simulink model "QuadRotor_PID_Simulink3d"  (R2014a)
settings: Solver=ode45  StartTime=0.0  StopTime=inf
PreLoadFcn:
  | load CommandsBus
model workspace (MAT data in the model file):
  thrustConstant = Simulink.Parameter
  thrustConstant.Value = -0.001
  thrustConstant.Description = '-0.004'
  thrustConstant.DataType = 'double'
  torqueConstant = Simulink.Parameter
  torqueConstant.Value = -4e-05
  torqueConstant.DataType = 'auto'
undefined symbols (not defined in the file or in its folder): X, Y, Z
libraries: sm_lib x829, nesl_utility x156, simulink x12, fl_lib x4, vrlib x4, aerolibtransform2 x1
(part 1 of 18)
settings Model: Creator=Leonardo  LastModifiedBy=jsustare
settings DataIOCC: OutputTimes=(1:900)*1/30
settings OptimizationCC: BlockReduction=off
settings DebuggingCC: UnderspecifiedInitializationDetection=Classic
settings ExplorerConfigSet: InternalSimMechanicsExplorerSettings="<ExplorerConfiguration><canonicalview>default</canonicalview><TilePanel><TileInfo><Tiles Columns=\"1\" Count=\"1\" Rows=\"1\"><Column Left=\"2\" Weight=\"1\"/><Column Left=\"1104\"/><Row Top=\"2\" Weight=\"1\"/><Row Top=\"593\"/><Tile Height=\"1\" Width=\"1\" X=\"0\" Y=\"0\"/></Tiles></TileInfo><SceneInfo><SceneViewer><BGColor><R>0.60000002384185791</R><G>0.60000002384185791</G><B>0.60000002384185791</B></BGColor><Camera><Position><X>6.7360474591593813e-05</X><Y>0.35928378687683804</Y><Z>0.81921140974164575</Z></Position><Center><X>6.7360474591593813e-05</X><Y>0.35928378687683804</Y><Z>0</Z></Center><Up><X>0</X><Y>1</Y><Z>-0</Z></Up><Left>-0.51821660457900831</Left><Right>0.51821660457900831</Right><Bottom>-0.41561021241290713</Bottom><Top>0.41561021241290713</Top></Camera></SceneViewer></SceneInfo></TilePanel></ExplorerConfiguration>"

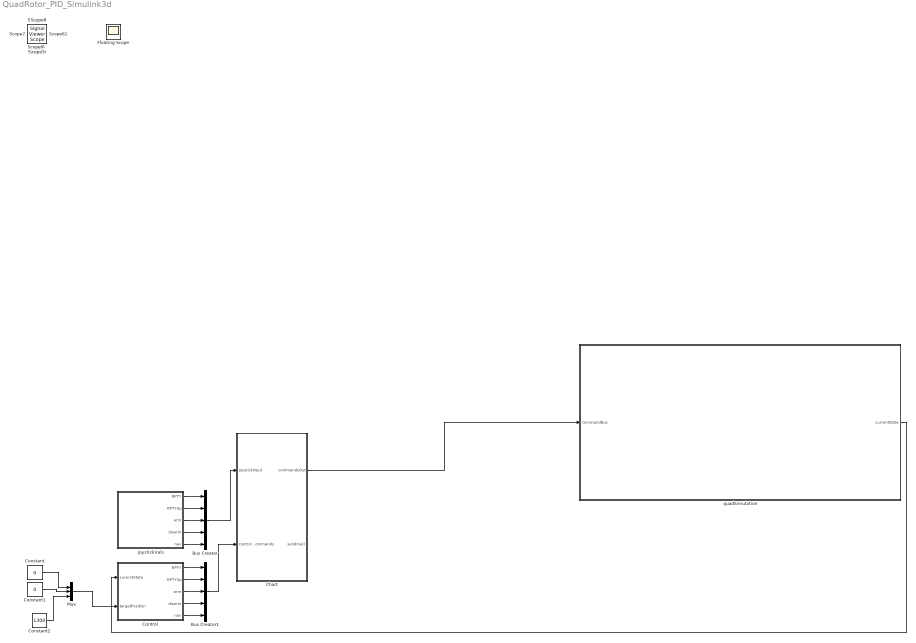
== system QuadRotor_PID_Simulink3d ==
  Bus Creator : BusCreator  Inputs=5
  Bus Creator1 : BusCreator  Inputs=5  OutDataTypeStr=Bus: CommandsBus
  Chart : Stateflow chart  TreatAsAtomicUnit=on
  Constant : Constant  Value=0
  Constant1 : Constant  Value=0
  Constant2 : Constant  Value=1300
  Control : Subsystem
  Mux : Mux  Inputs=3
  joystickVals : Subsystem
  quadSimulation : Subsystem
  Floating Scope : Scope
      settings: Floating=on  YMin=-0.125  YMax=0.15  SaveName=ScopeData8
  Scope{,1..4} (5 alike) : SignalViewerScope  IOType=viewer  RefreshTime=0.035000
      Scope settings: YMin=-0.7  YMax=0.1  SaveName=ScopeData4
      Scope1 settings: YMin=5.81481  YMax=6.42689
      Scope3 settings: YMin=-2.5  YMax=20  SaveName=ScopeData2
      Scope4 settings: YMin=0.0225  YMax=0.05  SaveName=ScopeData3
  Scope10 : SignalViewerScope  IOType=viewer  NumInputPorts=3  LegendLocations=|  RefreshTime=0.035000
      | 0.58116     0.90774     0.17375    0.026284
      | 0.69749     0.61398     0.23192    0.026284
      | 0.67959         0.3     0.24981    0.026284
      settings: ShowLegends=on  YMin=-0.09~-400~-1  YMax=0.1~450~1  SaveName=ScopeData10
  Scope11 : SignalViewerScope  IOType=viewer  NumInputPorts=3  RefreshTime=0.035000
      settings: YMin=-0.5~-750~-1  YMax=9.5~750~1  SaveName=ScopeData11
  Scope5 : SignalViewerScope  IOType=viewer  NumInputPorts=2  RefreshTime=0.035000
      settings: YMin=-55~-5  YMax=5~5  SaveName=ScopeData5
  Scope6 : SignalViewerScope  IOType=viewer  NumInputPorts=4  RefreshTime=0.035000
      settings: YMin=-35~-35~-550~-4  YMax=10~10~50~2  SaveName=ScopeData9
  Scope7 : SignalViewerScope  IOType=viewer  NumInputPorts=3  RefreshTime=0.035000
      settings: YMin=-0.1~-10~0  YMax=1.1~10~1  SaveName=ScopeData6
  Scope8 : SignalViewerScope  IOType=viewer  NumInputPorts=2  RefreshTime=0.035000
      settings: YMin=-125~-10  YMax=150~12.5  SaveName=ScopeData7
  Scope9 : SignalViewerScope  IOType=viewer  NumInputPorts=3  RefreshTime=0.035000
      settings: YMin=-0.1~-10~0  YMax=1.1~10~1  SaveName=ScopeData8
  wires:
  joystickVals/4(disarm) -> Bus Creator/4
  joystickVals/3(arm) -> Bus Creator/3
  joystickVals/5(nav) -> Bus Creator/5
  Bus Creator/1 -> Chart/1(joystickInput)
  Control/5(nav) -> Bus Creator1/5
  Control/4(disarm) -> Bus Creator1/4
  Control/3(arm) -> Bus Creator1/3
  Control/2(RPTYUp) -> Bus Creator1/2
  Control/1(RPTY) -> Bus Creator1/1
  Bus Creator1/1 -> Chart/2(controlCommands)
  joystickVals/1(RPTY) -> Bus Creator/1
  joystickVals/2(RPTYUp) -> Bus Creator/2
  Chart/1(commandsOut) -> quadSimulation/1(commandBus)
  quadSimulation/1(currentState) -> Control/1(curerntState)
  Constant/1 -> Mux/1
  Constant1/1 -> Mux/2
  Constant2/1 -> Mux/3
  Mux/1 -> Control/2(targetPosition)

== system QuadRotor_PID_Simulink3d/Control ==
  curerntState : Inport
  targetPosition : Inport  Port=2
  Band-Limited White Noise : simulink/Sources/Band-Limited White Noise  Cov=0.00005  Ts=0.1  seed=[23341]
  Band-Limited White Noise1 : simulink/Sources/Band-Limited White Noise  Cov=0.00005  Ts=0.1  seed=[23341]
  Band-Limited White Noise2 : simulink/Sources/Band-Limited White Noise  Cov=0.00005  Ts=0.1  seed=[23341]
  Constant : Constant  OutDataTypeStr=boolean
  Demux : Demux  Outputs=6
  Detect Change : simulink/Logic and Bit Operations/Detect Change  vinit=0  InputProcessing=Inherited  OutDataTypeStr=boolean
  Logical Operator : Logic  Operator=OR  Inputs=1  AllPortsSameDT=off  OutDataTypeStr=boolean
  Mux : Mux
  Sum : Sum  Inputs=|++
  Sum1 : Sum  Inputs=|++
  Sum2 : Sum  Inputs=|++
  failsafes : Subsystem
  positionControl : Subsystem
  RPTY : Outport
  RPTYUp : Outport  Port=2
  arm : Outport  Port=3
  disarm : Outport  Port=4
  nav : Outport  Port=5
  wires:
  Demux/5 -> Sum/2
  Demux/6 -> Sum1/2
  Demux/3 -> Sum2/2
  positionControl/1(R) -> Mux/1
  positionControl/2(P) -> Mux/2
  positionControl/4(Thrust) -> Mux/3
  positionControl/3(targetYaw) -> Mux/4
  Mux/1 -> Detect Change/1, RPTY/1
  Detect Change/1 -> Logical Operator/1
  Logical Operator/1 -> RPTYUp/1
  Constant/1 -> nav/1
  targetPosition/1 -> positionControl/4(targetPos)
  failsafes/1(arm) -> arm/1
  failsafes/2(disarm) -> disarm/1
  curerntState/1 -> Demux/1
  Band-Limited White Noise/1 -> Sum/1
  Sum/1 -> positionControl/1(X)
  Band-Limited White Noise1/1 -> Sum1/1
  Sum1/1 -> positionControl/2(Y)
  Band-Limited White Noise2/1 -> Sum2/1
  Sum2/1 -> positionControl/3(Heading)

== system QuadRotor_PID_Simulink3d/joystickVals ==
  Constant1 : Constant  Value=0  OutDataTypeStr=boolean
  Constant2 : Constant  Value=0  OutDataTypeStr=boolean
  Constant3 : Constant  Value=1500
  Constant4 : Constant  Value=1500
  Constant5 : Constant  Value=1059
  Constant6 : Constant  Value=1500
  Constant7 : Constant  OutDataTypeStr=boolean
  Detect Change : simulink/Logic and Bit Operations/Detect Change  vinit=0  InputProcessing=Inherited  OutDataTypeStr=boolean
  Logical Operator : Logic  Operator=OR  Inputs=1  AllPortsSameDT=off  OutDataTypeStr=boolean
  Mux : Mux
  RPTY : Outport
  RPTYUp : Outport  Port=2
  arm : Outport  Port=3
  disarm : Outport  Port=4
  nav : Outport  Port=5
  wires:
  Constant3/1 -> Mux/2
  Constant4/1 -> Mux/1
  Constant5/1 -> Mux/3
  Constant6/1 -> Mux/4
  Mux/1 -> RPTY/1, Detect Change/1  "RPTY"
  Detect Change/1 -> Logical Operator/1
  Logical Operator/1 -> RPTYUp/1  "RPTYUp"
  Constant1/1 -> arm/1  "arm"
  Constant2/1 -> disarm/1  "disarm"
  Constant7/1 -> nav/1  "nav"

== system QuadRotor_PID_Simulink3d/quadSimulation ==
  note: Pitch (Motor A,C)
      | Roll (Motor B,D)
      | Altitude(A,B,C,D)
      | Yaw (Unbalance A/C B/D)
  commandBus : Inport
  Controller : Subsystem
  Demux : Demux
  GetErrors : Subsystem
  Mux : Mux  Inputs=6
  Mux2 : Mux
  Plant_Quad_Base : Subsystem  Variant=on  OverrideUsingVariant=Quad_6DOF
  Rate Transition : RateTransition
  Scope6 : Scope  NumInputPorts=4
      settings: YMin=-5~-5~-5~-5  YMax=5~5~5~5  SaveName=ScopeData6
  SpdMin2Rotors : Constant  Value=0.058
  Vizualize Signals : Subsystem
  Vizualize Simulink 3d : Subsystem
  converting : Subsystem
  currentState : Outport
  wires:
  Plant_Quad_Base/1(Roll) -> Mux/1  "Roll"
  Plant_Quad_Base/2(Pitch) -> Mux/2  "Pitch"
  Plant_Quad_Base/3(Yaw) -> Mux/3  "Yaw"
  Plant_Quad_Base/4(Altitude) -> Mux/4  "Altitude"
  Controller/2(Act_B) -> Plant_Quad_Base/2(spdMotorB)
  Controller/3(Act_C) -> Plant_Quad_Base/3(spdMotorC)
  Controller/1(Act_A) -> Plant_Quad_Base/1(spdMotorA)
  Controller/4(Act_D) -> Plant_Quad_Base/4(spdMotorD)
  SpdMin2Rotors/1 -> Controller/1(Ref_Spd_Min)
  Demux/1 -> Scope6/1, Controller/2(Err_Roll)  "Err_Roll"
  Demux/2 -> Scope6/2, Controller/3(Err_Pitch)  "Err_Pitch"
  Demux/3 -> Scope6/3, Controller/4(Err_Yaw)  "Err_Yaw"
  Demux/4 -> Scope6/4, Controller/5(Err_Alt)  "Err_Alt"
  Plant_Quad_Base/5(X) -> Mux/5  "X"
  Plant_Quad_Base/6(Y) -> Mux/6  "Y"
  Rate Transition/1 -> GetErrors/1(References)
  GetErrors/1(Errors) -> Demux/1
  Mux2/1 -> Rate Transition/1
  Mux/1 -> GetErrors/2(Outputs), currentState/1
  commandBus/1 -> converting/1(In1)
  converting/1(Out1) -> Mux2/1
  converting/2(Out2) -> Mux2/2
  converting/3(Out3) -> Mux2/3
  converting/4(Out4) -> Mux2/4

== system QuadRotor_PID_Simulink3d/Control/failsafes ==
  Constant1 : Constant  Value=0  OutDataTypeStr=boolean
  arm : Outport
  disarm : Outport  Port=2
  wires:
  Constant1/1 -> disarm/1, arm/1

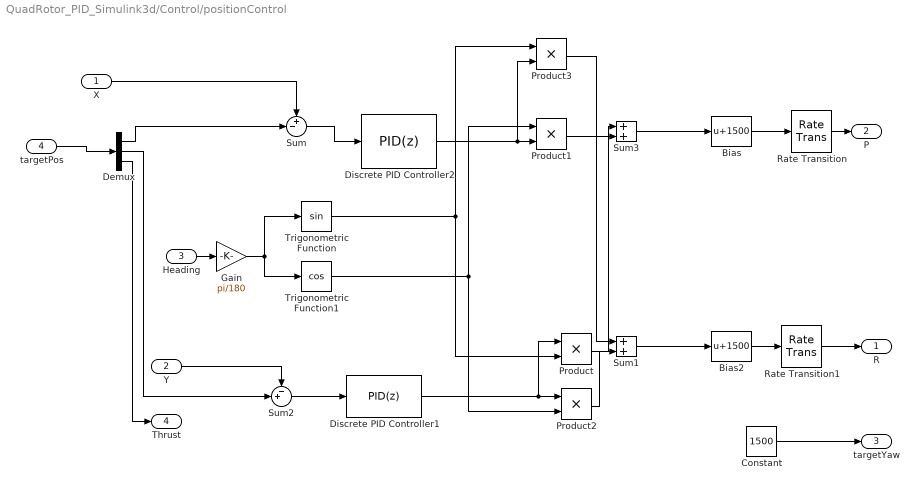
== system QuadRotor_PID_Simulink3d/Control/positionControl ==
  X : Inport
  Y : Inport  Port=2
  Heading : Inport  Port=3
  targetPos : Inport  Port=4
  Bias : Bias  Bias=1500
  Bias2 : Bias  Bias=1500
  Constant : Constant  Value=1500
  Demux : Demux  Outputs=3
  Discrete PID Controller1 : simulink/Continuous/PID Controller  Controller=PID  TimeDomain=Discrete-time  SampleTime=0.1  IntegratorMethod=Trapezoidal  FilterMethod=Trapezoidal  Form=Parallel  P=300  I=0  D=250  N=100  InitialConditionSource=internal  InitialConditionForIntegrator=0  InitialConditionForFilter=0  ExternalReset=none  ZeroCross=off  LimitOutput=on  UpperSaturationLimit=500  LowerSaturationLimit=-500  LinearizeAsGain=off  AntiWindupMode=clamping  Kb=1  TrackingMode=off  Kt=1  PParamMin=[]  PParamMax=[]  IParamMin=[]  IParamMax=[]  DParamMin=[]  DParamMax=[]  NParamMin=[]  NParamMax=[]  KbParamMin=[]  KbParamMax=[]  KtParamMin=[]  KtParamMax=[]  POutMin=[]  POutMax=[]  IOutMin=[]  IOutMax=[]  DOutMin=[]  DOutMax=[]  NOutMin=[]  NOutMax=[]  KbOutMin=[]  KbOutMax=[]  KtOutMin=[]  KtOutMax=[]  IntegratorOutMin=[]  IntegratorOutMax=[]  FilterOutMin=[]  FilterOutMax=[]  SumOutMin=[]  SumOutMax=[]  SumI1OutMin=[]  SumI1OutMax=[]  SumI2OutMin=[]  SumI2OutMax=[]  SumI3OutMin=[]  SumI3OutMax=[]  SumDOutMin=[]  SumDOutMax=[]  SaturationOutMin=[]  SaturationOutMax=[]  IntegratorContinuousStateAttributes=''  IntegratorStateMustResolveToSignalObject=off  IntegratorRTWStateStorageClass=Auto  FilterContinuousStateAttributes=''  FilterStateMustResolveToSignalObject=off  FilterRTWStateStorageClass=Auto
  Discrete PID Controller2 : simulink/Continuous/PID Controller  Controller=PID  TimeDomain=Discrete-time  SampleTime=0.1  IntegratorMethod=Trapezoidal  FilterMethod=Trapezoidal  Form=Parallel  P=300  I=0  D=250  N=100  InitialConditionSource=internal  InitialConditionForIntegrator=0  InitialConditionForFilter=0  ExternalReset=none  ZeroCross=off  LimitOutput=on  UpperSaturationLimit=500  LowerSaturationLimit=-500  LinearizeAsGain=off  AntiWindupMode=clamping  Kb=1  TrackingMode=off  Kt=1  PParamMin=[]  PParamMax=[]  IParamMin=[]  IParamMax=[]  DParamMin=[]  DParamMax=[]  NParamMin=[]  NParamMax=[]  KbParamMin=[]  KbParamMax=[]  KtParamMin=[]  KtParamMax=[]  POutMin=[]  POutMax=[]  IOutMin=[]  IOutMax=[]  DOutMin=[]  DOutMax=[]  NOutMin=[]  NOutMax=[]  KbOutMin=[]  KbOutMax=[]  KtOutMin=[]  KtOutMax=[]  IntegratorOutMin=[]  IntegratorOutMax=[]  FilterOutMin=[]  FilterOutMax=[]  SumOutMin=[]  SumOutMax=[]  SumI1OutMin=[]  SumI1OutMax=[]  SumI2OutMin=[]  SumI2OutMax=[]  SumI3OutMin=[]  SumI3OutMax=[]  SumDOutMin=[]  SumDOutMax=[]  SaturationOutMin=[]  SaturationOutMax=[]  IntegratorContinuousStateAttributes=''  IntegratorStateMustResolveToSignalObject=off  IntegratorRTWStateStorageClass=Auto  FilterContinuousStateAttributes=''  FilterStateMustResolveToSignalObject=off  FilterRTWStateStorageClass=Auto
  Gain : Gain  Gain=pi/180
  Product{,1..3} (4 alike) : Product
  Rate Transition : RateTransition
  Rate Transition1 : RateTransition
  Sum : Sum  Inputs=+-|
  Sum1 : Sum
  Sum2 : Sum  Inputs=-+|
  Sum3 : Sum
  Trigonometric Function : Trigonometry
  Trigonometric Function1 : Trigonometry  Operator=cos
  R : Outport
  P : Outport  Port=2
  targetYaw : Outport  Port=3
  Thrust : Outport  Port=4
  wires:
  Sum/1 -> Discrete PID Controller2/1
  Heading/1 -> Gain/1
  Gain/1 -> Trigonometric Function/1, Trigonometric Function1/1
  Discrete PID Controller1/1 -> Product/1, Product2/1
  Trigonometric Function/1 -> Product/2, Product3/1
  Discrete PID Controller2/1 -> Product3/2, Product1/2
  Trigonometric Function1/1 -> Product2/2, Product1/1
  Product1/1 -> Sum3/2
  Product2/1 -> Sum1/2
  Sum3/1 -> Bias/1
  Product3/1 -> Sum1/1
  targetPos/1 -> Demux/1
  Demux/1 -> Sum/2
  Constant/1 -> targetYaw/1
  Rate Transition/1 -> P/1
  Rate Transition1/1 -> R/1
  Bias/1 -> Rate Transition/1
  Demux/3 -> Thrust/1
  Product/1 -> Sum3/1
  Sum1/1 -> Bias2/1
  Bias2/1 -> Rate Transition1/1
  Sum2/1 -> Discrete PID Controller1/1
  Demux/2 -> Sum2/2
  Y/1 -> Sum2/1
  X/1 -> Sum/1

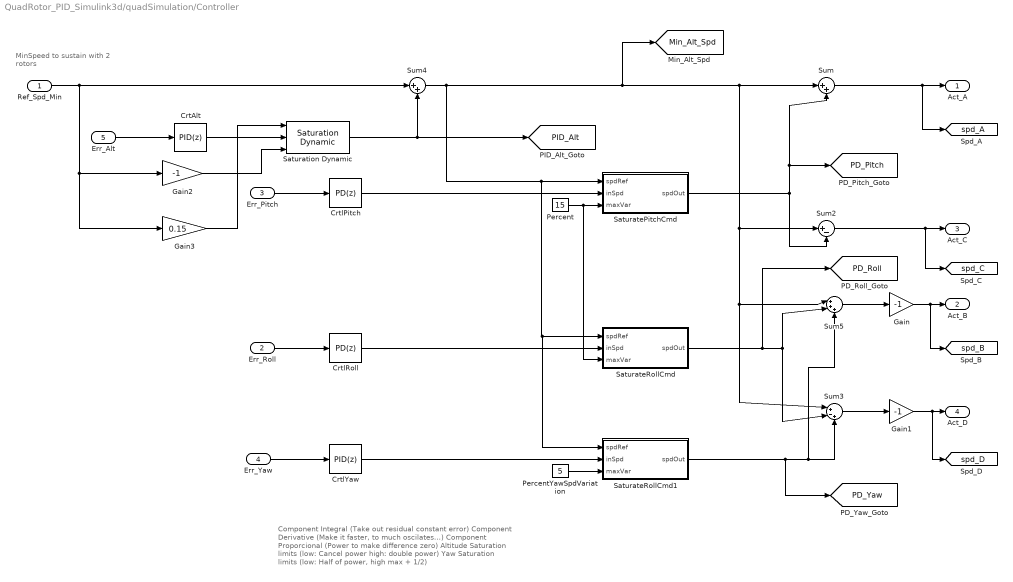
== system QuadRotor_PID_Simulink3d/quadSimulation/Controller ==
  note: MinSpeed to sustain with 2
      | rotors
  note: Component Integral (Take out residual constant error)
      | Component Derivative (Make it faster, to much oscilates...)
      | Component Proporcional (Power to make difference zero)
      |
      | Altitude
      | Saturation limits (low: Cancel power high: double power)
      |
      | Yaw
      | Saturation limits (low: Half of power, high max + 1/2)
  Ref_Spd_Min : Inport
  Err_Roll : Inport  Port=2
  Err_Pitch : Inport  Port=3
  Err_Yaw : Inport  Port=4
  Err_Alt : Inport  Port=5
  CrtAlt : simulink/Continuous/PID Controller  Controller=PID  TimeDomain=Discrete-time  SampleTime=0.001  IntegratorMethod=Forward Euler  FilterMethod=Forward Euler  Form=Parallel  P=0.4  I=0.01  D=0.2  N=100  InitialConditionSource=internal  InitialConditionForIntegrator=0  InitialConditionForFilter=0  ExternalReset=none  LimitOutput=off  UpperSaturationLimit=0.116  LowerSaturationLimit=-0.116  LinearizeAsGain=off  AntiWindupMode=none  Kb=1  TrackingMode=off  Kt=1  PParamMin=[]  PParamMax=[]  IParamMin=[]  IParamMax=[]  DParamMin=[]  DParamMax=[]  NParamMin=[]  NParamMax=[]  KbParamMin=[]  KbParamMax=[]  KtParamMin=[]  KtParamMax=[]  POutMin=[]  POutMax=[]  IOutMin=[]  IOutMax=[]  DOutMin=[]  DOutMax=[]  NOutMin=[]  NOutMax=[]  KbOutMin=[]  KbOutMax=[]  KtOutMin=[]  KtOutMax=[]  IntegratorOutMin=[]  IntegratorOutMax=[]  FilterOutMin=[]  FilterOutMax=[]  SumOutMin=[]  SumOutMax=[]  SumI1OutMin=[]  SumI1OutMax=[]  SumI2OutMin=[]  SumI2OutMax=[]  SumI3OutMin=[]  SumI3OutMax=[]  SumDOutMin=[]  SumDOutMax=[]  SaturationOutMin=[]  SaturationOutMax=[]  IntegratorContinuousStateAttributes=''  IntegratorStateMustResolveToSignalObject=off  IntegratorRTWStateStorageClass=Auto  FilterContinuousStateAttributes=''  FilterStateMustResolveToSignalObject=off  FilterRTWStateStorageClass=Auto
  CrtlPitch : simulink/Continuous/PID Controller  Controller=PD  TimeDomain=Discrete-time  SampleTime=0.001  IntegratorMethod=Forward Euler  FilterMethod=Forward Euler  Form=Parallel  P=0.01  I=0  D=0.001  N=100  InitialConditionSource=internal  InitialConditionForIntegrator=0  InitialConditionForFilter=0  ExternalReset=none  LimitOutput=off  UpperSaturationLimit=+Inf  LowerSaturationLimit=0  LinearizeAsGain=off  AntiWindupMode=none  Kb=1  TrackingMode=off  Kt=1  PParamMin=[]  PParamMax=[]  IParamMin=[]  IParamMax=[]  DParamMin=[]  DParamMax=[]  NParamMin=[]  NParamMax=[]  KbParamMin=[]  KbParamMax=[]  KtParamMin=[]  KtParamMax=[]  POutMin=[]  POutMax=[]  IOutMin=[]  IOutMax=[]  DOutMin=[]  DOutMax=[]  NOutMin=[]  NOutMax=[]  KbOutMin=[]  KbOutMax=[]  KtOutMin=[]  KtOutMax=[]  IntegratorOutMin=[]  IntegratorOutMax=[]  FilterOutMin=[]  FilterOutMax=[]  SumOutMin=[]  SumOutMax=[]  SumI1OutMin=[]  SumI1OutMax=[]  SumI2OutMin=[]  SumI2OutMax=[]  SumI3OutMin=[]  SumI3OutMax=[]  SumDOutMin=[]  SumDOutMax=[]  SaturationOutMin=[]  SaturationOutMax=[]  IntegratorContinuousStateAttributes=''  IntegratorStateMustResolveToSignalObject=off  IntegratorRTWStateStorageClass=Auto  FilterContinuousStateAttributes=''  FilterStateMustResolveToSignalObject=off  FilterRTWStateStorageClass=Auto
  CrtlRoll : simulink/Continuous/PID Controller  Controller=PD  TimeDomain=Discrete-time  SampleTime=0.001  IntegratorMethod=Forward Euler  FilterMethod=Forward Euler  Form=Parallel  P=0.01  I=0  D=0.001  N=100  InitialConditionSource=internal  InitialConditionForIntegrator=0  InitialConditionForFilter=0  ExternalReset=none  LimitOutput=off  UpperSaturationLimit=0.058  LowerSaturationLimit=-0.058  LinearizeAsGain=off  AntiWindupMode=none  Kb=1  TrackingMode=off  Kt=1  PParamMin=[]  PParamMax=[]  IParamMin=[]  IParamMax=[]  DParamMin=[]  DParamMax=[]  NParamMin=[]  NParamMax=[]  KbParamMin=[]  KbParamMax=[]  KtParamMin=[]  KtParamMax=[]  POutMin=[]  POutMax=[]  IOutMin=[]  IOutMax=[]  DOutMin=[]  DOutMax=[]  NOutMin=[]  NOutMax=[]  KbOutMin=[]  KbOutMax=[]  KtOutMin=[]  KtOutMax=[]  IntegratorOutMin=[]  IntegratorOutMax=[]  FilterOutMin=[]  FilterOutMax=[]  SumOutMin=[]  SumOutMax=[]  SumI1OutMin=[]  SumI1OutMax=[]  SumI2OutMin=[]  SumI2OutMax=[]  SumI3OutMin=[]  SumI3OutMax=[]  SumDOutMin=[]  SumDOutMax=[]  SaturationOutMin=[]  SaturationOutMax=[]  IntegratorContinuousStateAttributes=''  IntegratorStateMustResolveToSignalObject=off  IntegratorRTWStateStorageClass=Auto  FilterContinuousStateAttributes=''  FilterStateMustResolveToSignalObject=off  FilterRTWStateStorageClass=Auto
  CrtlYaw : simulink/Continuous/PID Controller  Controller=PID  TimeDomain=Discrete-time  SampleTime=0.001  IntegratorMethod=Forward Euler  FilterMethod=Forward Euler  Form=Parallel  P=-0.0001  I=0  D=-0.0001  N=100  InitialConditionSource=internal  InitialConditionForIntegrator=0  InitialConditionForFilter=0  ExternalReset=none  LimitOutput=off  UpperSaturationLimit=0.01  LowerSaturationLimit=-0.01  LinearizeAsGain=off  AntiWindupMode=none  Kb=1  TrackingMode=off  Kt=1  PParamMin=[]  PParamMax=[]  IParamMin=[]  IParamMax=[]  DParamMin=[]  DParamMax=[]  NParamMin=[]  NParamMax=[]  KbParamMin=[]  KbParamMax=[]  KtParamMin=[]  KtParamMax=[]  POutMin=[]  POutMax=[]  IOutMin=[]  IOutMax=[]  DOutMin=[]  DOutMax=[]  NOutMin=[]  NOutMax=[]  KbOutMin=[]  KbOutMax=[]  KtOutMin=[]  KtOutMax=[]  IntegratorOutMin=[]  IntegratorOutMax=[]  FilterOutMin=[]  FilterOutMax=[]  SumOutMin=[]  SumOutMax=[]  SumI1OutMin=[]  SumI1OutMax=[]  SumI2OutMin=[]  SumI2OutMax=[]  SumI3OutMin=[]  SumI3OutMax=[]  SumDOutMin=[]  SumDOutMax=[]  SaturationOutMin=[]  SaturationOutMax=[]  IntegratorContinuousStateAttributes=''  IntegratorStateMustResolveToSignalObject=off  IntegratorRTWStateStorageClass=Auto  FilterContinuousStateAttributes=''  FilterStateMustResolveToSignalObject=off  FilterRTWStateStorageClass=Auto
  Gain : Gain  Gain=-1
  Gain1 : Gain  Gain=-1
  Gain2 : Gain  Gain=-1
  Gain3 : Gain  Gain=0.15
  Percent : Constant  Value=15
  PercentYawSpdVariation : Constant  Value=5
  SaturatePitchCmd : MATLAB Function  TreatAsAtomicUnit=on
  SaturateRollCmd : MATLAB Function  TreatAsAtomicUnit=on
  SaturateRollCmd1 : MATLAB Function  TreatAsAtomicUnit=on
  Saturation Dynamic : simulink/Discontinuities/Saturation Dynamic  OutMin=[]  OutMax=[]  OutDataTypeStr=Inherit: Same as second input  OutDataType=fixdt(1, 16)  OutScaling=2^-10  DoSatur=off
  Sum : Sum  Inputs=|++
  Sum2 : Sum  Inputs=|+-
  Sum3 : Sum  Inputs=|+-+
  Sum4 : Sum  Inputs=|++
  Sum5 : Sum  Inputs=|+++
  Act_A : Outport
  Act_B : Outport  Port=2
  Act_C : Outport  Port=3
  Act_D : Outport  Port=4
  tag scope: Min_Alt_Spd=global, PD_Pitch=global, PD_Roll=global, PD_Yaw=global, PID_Alt=global, spd_A=global, spd_B=global, spd_C=global, spd_D=global
  wires:
  Err_Alt/1 -> CrtAlt/1
  Ref_Spd_Min/1 -> Sum4/1, Gain3/1, Gain2/1
  Err_Yaw/1 -> CrtlYaw/1
  Err_Pitch/1 -> CrtlPitch/1
  Err_Roll/1 -> CrtlRoll/1
  Sum5/1 -> Gain/1
  Sum3/1 -> Gain1/1
  Gain/1 -> [spd_B], Act_B/1
  Gain1/1 -> [spd_D], Act_D/1
  Sum/1 -> [spd_A], Act_A/1
  Sum2/1 -> [spd_C], Act_C/1
  Sum4/1 -> SaturateRollCmd1/1(spdRef), SaturateRollCmd/1(spdRef), SaturatePitchCmd/1(spdRef), [Min_Alt_Spd], Sum2/1, Sum5/1, Sum3/1, Sum/1
  SaturatePitchCmd/1(spdOut) -> [PD_Pitch], Sum/2, Sum2/2
  Percent/1 -> SaturateRollCmd/3(maxVar), SaturatePitchCmd/3(maxVar)
  SaturateRollCmd/1(spdOut) -> [PD_Roll], Sum3/2, Sum5/2
  PercentYawSpdVariation/1 -> SaturateRollCmd1/3(maxVar)
  SaturateRollCmd1/1(spdOut) -> [PD_Yaw], Sum5/3, Sum3/3
  CrtAlt/1 -> Saturation Dynamic/2
  Gain2/1 -> Saturation Dynamic/3
  Gain3/1 -> Saturation Dynamic/1
  CrtlYaw/1 -> SaturateRollCmd1/2(inSpd)
  CrtlPitch/1 -> SaturatePitchCmd/2(inSpd)
  CrtlRoll/1 -> SaturateRollCmd/2(inSpd)
  Saturation Dynamic/1 -> [PID_Alt], Sum4/2

== system QuadRotor_PID_Simulink3d/quadSimulation/GetErrors ==
  References : Inport
  Outputs : Inport  Port=2
  Demux : Demux
  Demux1 : Demux  Outputs=6
  Mux : Mux
  Scope : Scope  NumInputPorts=4
      settings: YMin=-7.5~-7.5~-0.2~-2  YMax=12.5~7.5~0.2~2  SaveName=ScopeData5
  Sum{,1..2,10} (4 alike) : Sum  Inputs=|+-
  Errors : Outport
  tag scope: Ref_Alt=global, Ref_Alt_Err=global, Ref_Pitch=global, Ref_Pitch_Err=global, Ref_Roll=global, Ref_Roll_Err=global, Ref_Yaw=global, Ref_Yaw_Err=global
  wires:
  References/1 -> Demux/1
  Outputs/1 -> Demux1/1
  Demux/1 -> [Ref_Roll], Sum10/1  "Ref_Roll"
  Demux1/1 -> Sum10/2  "Roll"
  Demux/2 -> [Ref_Pitch], Sum/1  "Ref_Pitch"
  Demux/3 -> [Ref_Yaw], Sum1/1  "Ref_Yaw"
  Demux1/2 -> Sum/2  "Pitch"
  Demux1/3 -> Sum1/2  "Yaw"
  Demux/4 -> [Ref_Alt], Sum2/1  "Ref_Alt"
  Demux1/4 -> Sum2/2  "Altitude"
  Sum2/1 -> [Ref_Alt_Err], Scope/4, Mux/4  "Err_Alt"
  Sum1/1 -> [Ref_Yaw_Err], Scope/3, Mux/3  "Err_Yaw"
  Sum/1 -> [Ref_Pitch_Err], Scope/2, Mux/2  "Err_Pitch"
  Sum10/1 -> [Ref_Roll_Err], Scope/1, Mux/1  "Err_Roll"
  Mux/1 -> Errors/1

== system QuadRotor_PID_Simulink3d/quadSimulation/Plant_Quad_Base ==
  note: 1) Only subsystems can be added as variant choices at this level
      | 2) Blocks cannot be connected at this level as connectivity is
      | automatically determined at simulation, based on the active variant
  spdMotorA : Inport
  spdMotorB : Inport  Port=2
  spdMotorC : Inport  Port=3
  spdMotorD : Inport  Port=4
  Quad_6Dof : Subsystem  VariantControl=Quad_6DOF
  Quad_Altitude : Subsystem  VariantControl=Quad_A
  Quad_Pitch : Subsystem  VariantControl=Quad_P
  Quad_Roll : Subsystem  VariantControl=Quad_R
  Quad_Roll_Pitch_Yaw : Subsystem  VariantControl=Quad_R_P_Y
  Quad_Roll_Pitch_Yaw_Altitude : Subsystem  VariantControl=Quad_R_P_Y_A
  Quad_Yaw : Subsystem  VariantControl=Quad_Y
  Quad_Yaw_Altitude : Subsystem  VariantControl=Quad_Y_A
  Roll : Outport
  Pitch : Outport  Port=2
  Yaw : Outport  Port=3
  Altitude : Outport  Port=4
  X : Outport  Port=5
  Y : Outport  Port=6

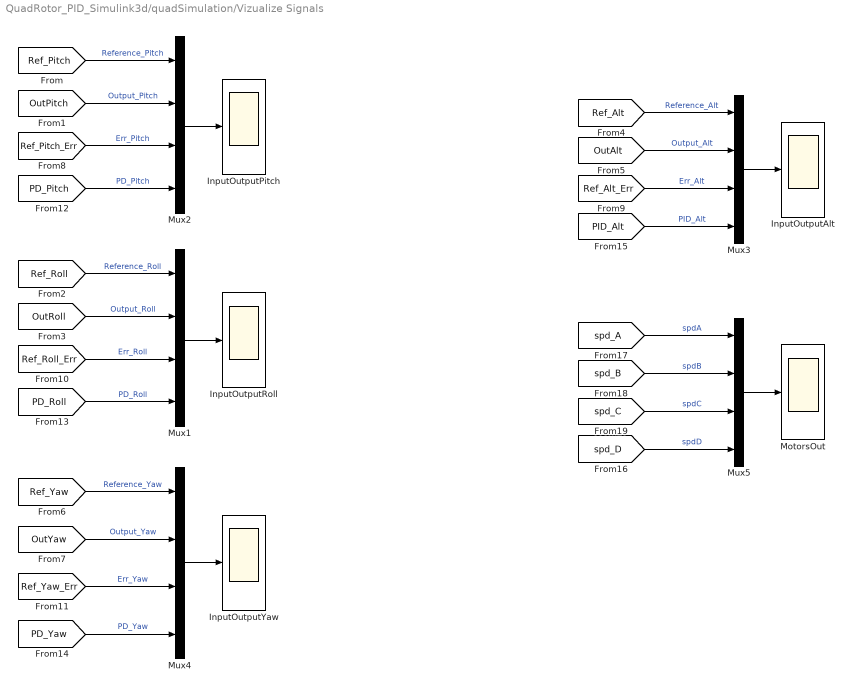
== system QuadRotor_PID_Simulink3d/quadSimulation/Vizualize Signals ==
  InputOutputAlt : Scope
      settings: ShowLegends=on  TimeRange=30  YMin=-900  YMax=900  SaveName=ScopeData3
  InputOutputPitch : Scope
      settings: ShowLegends=on  YMin=-90  YMax=140
  InputOutputRoll : Scope
      settings: ShowLegends=on  SaveName=ScopeData2
  InputOutputYaw : Scope
      settings: ShowLegends=on  SaveName=ScopeData4
  MotorsOut : Scope
      settings: ShowLegends=on  TimeRange=30  YMin=-900  YMax=900
  Mux{1..5} (5 alike) : Mux
  wires:
  Mux2/1 -> InputOutputPitch/1
  [OutPitch] -> Mux2/2  "Output_Pitch"
  [Ref_Pitch] -> Mux2/1  "Reference_Pitch"
  Mux1/1 -> InputOutputRoll/1
  [OutRoll] -> Mux1/2  "Output_Roll"
  [Ref_Roll] -> Mux1/1  "Reference_Roll"
  Mux3/1 -> InputOutputAlt/1
  [OutAlt] -> Mux3/2  "Output_Alt"
  [Ref_Alt] -> Mux3/1  "Reference_Alt"
  Mux4/1 -> InputOutputYaw/1
  [OutYaw] -> Mux4/2  "Output_Yaw"
  [Ref_Yaw] -> Mux4/1  "Reference_Yaw"
  [Ref_Pitch_Err] -> Mux2/3  "Err_Pitch"
  [Ref_Alt_Err] -> Mux3/3  "Err_Alt"
  [Ref_Roll_Err] -> Mux1/3  "Err_Roll"
  [Ref_Yaw_Err] -> Mux4/3  "Err_Yaw"
  [PD_Pitch] -> Mux2/4  "PD_Pitch"
  [PD_Roll] -> Mux1/4  "PD_Roll"
  [PD_Yaw] -> Mux4/4  "PD_Yaw"
  [PID_Alt] -> Mux3/4  "PID_Alt"
  Mux5/1 -> MotorsOut/1
  [spd_B] -> Mux5/2  "spdB"
  [spd_A] -> Mux5/1  "spdA"
  [spd_C] -> Mux5/3  "spdC"
  [spd_D] -> Mux5/4  "spdD"

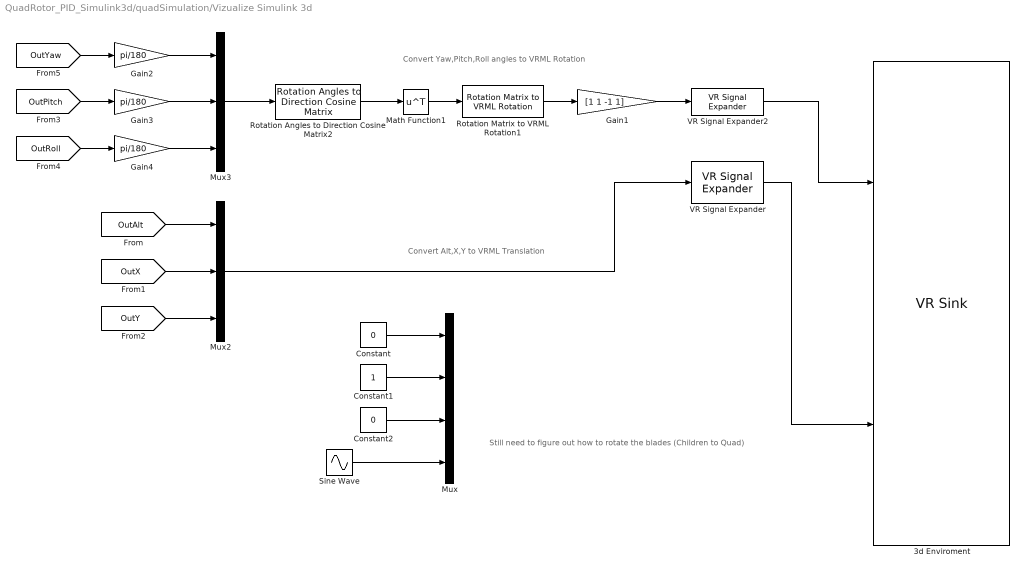
== system QuadRotor_PID_Simulink3d/quadSimulation/Vizualize Simulink 3d ==
  note: Still need to figure out how to rotate the blades (Children to Quad)
  note: Convert Alt,X,Y to VRML Translation
  note: Convert Yaw,Pitch,Roll angles to VRML Rotation
  3d Enviroment : vrlib/VR Sink  InstantiateOnLoad=on  SampleTime=0.1  ViewEnable=on  RemoteChange=off  RemoteView=off  FieldsWritten=Quadgroup.rotation.4.1.1.double#Quadgroup.translation.3.1.1.double  WorldFileName=Maya\simEnviroment.wrl  WorldDescription=simEnviroment  AutoView=off  VideoDimensions=[]  AllowVariableSize=off
  Constant : Constant  Value=0
  Constant1 : Constant
  Constant2 : Constant  Value=0
  Gain1 : Gain  Gain=[1 1 -1 1]
  Gain2 : Gain  Gain=pi/180
  Gain3 : Gain  Gain=pi/180
  Gain4 : Gain  Gain=pi/180
  Math Function1 : Math  Operator=transpose  SaturateOnIntegerOverflow=on
  Mux : Mux
  Mux2 : Mux  Inputs=3
  Mux3 : Mux  Inputs=3
  Rotation Angles to Direction Cosine Matrix2 : aerolibtransform2/Rotation Angles to Direction Cosine Matrix  rotationOrder=ZYX
  Rotation Matrix to VRML Rotation1 : vrlib/Utilities/Rotation Matrix to VRML Rotation  maxzero=1e-5
  Sine Wave : Sin  SampleTime=0
  VR Signal Expander : vrlib/VR Signal Expander  outwidth=3  outidx=[2 1 3]
  VR Signal Expander2 : vrlib/VR Signal Expander  outwidth=4  outidx=[1 3 2 4]
  wires:
  [OutPitch] -> Gain3/1
  Mux2/1 -> VR Signal Expander/1
  [OutY] -> Mux2/3
  [OutAlt] -> Mux2/1
  [OutX] -> Mux2/2
  Rotation Angles to Direction Cosine Matrix2/1 -> Math Function1/1
  Mux3/1 -> Rotation Angles to Direction Cosine Matrix2/1
  Rotation Matrix to VRML Rotation1/1 -> Gain1/1
  [OutYaw] -> Gain2/1
  Math Function1/1 -> Rotation Matrix to VRML Rotation1/1
  [OutRoll] -> Gain4/1
  Gain3/1 -> Mux3/2
  Gain4/1 -> Mux3/3
  Gain1/1 -> VR Signal Expander2/1
  Gain2/1 -> Mux3/1
  Constant/1 -> Mux/1
  Constant1/1 -> Mux/2
  Constant2/1 -> Mux/3
  Sine Wave/1 -> Mux/4
  VR Signal Expander2/1 -> 3d Enviroment/1
  VR Signal Expander/1 -> 3d Enviroment/2

== system QuadRotor_PID_Simulink3d/quadSimulation/converting ==
  In1 : Inport
  Bias : Bias  Bias=-1000
  Bias1 : Bias  Bias=-1500
  Bias2 : Bias  Bias=-1500
  Bias3 : Bias  Bias=-1500
  Bus Selector : BusSelector  OutputSignals=RPTY
  Demux1 : Demux
  Gain : Gain  Gain=2/500
  Gain1 : Gain  Gain=10/500
  Gain2 : Gain  Gain=180/500
  Gain3 : Gain  Gain=10/500
  Scope : Scope
      settings: YMin=5  SaveName=ScopeData7
  Scope1 : Scope
      settings: ShowLegends=on  YMin=-100  YMax=2000  SaveName=ScopeData9
  Out1 : Outport
  Out2 : Outport  Port=2
  Out3 : Outport  Port=3
  Out4 : Outport  Port=4
  wires:
  In1/1 -> Bus Selector/1
  Bias/1 -> Gain/1
  Bias3/1 -> Gain3/1
  Bias1/1 -> Gain2/1
  Demux1/2 -> Bias2/1
  Bus Selector/1 -> Scope1/1, Demux1/1  "<RPTY>"
  Gain3/1 -> Out1/1
  Demux1/1 -> Bias3/1
  Bias2/1 -> Gain1/1
  Gain1/1 -> Out2/1
  Demux1/3 -> Scope/1, Bias/1
  Gain/1 -> Out4/1
  Demux1/4 -> Bias1/1
  Gain2/1 -> Out3/1

== system QuadRotor_PID_Simulink3d/quadSimulation/Plant_Quad_Base/Quad_6Dof ==
  spdMotorA : Inport
  spdMotorB : Inport  Port=2
  spdMotorC : Inport  Port=3
  spdMotorD : Inport  Port=4
  BaseTestes : Subsystem
  Convert : Subsystem
  Convert1 : Subsystem
  Convert2 : Subsystem
  Convert3 : Subsystem
  QuadRotor : Subsystem
  Roll : Outport
  Pitch : Outport  Port=2
  Yaw : Outport  Port=3
  Altitude : Outport  Port=4
  X : Outport  Port=5
  Y : Outport  Port=6
  tag scope: OutAlt=global, OutPitch=global, OutRoll=global, OutX=global, OutY=global, OutYaw=global
  wires:
  spdMotorD/1 -> QuadRotor/4(motor_D)
  spdMotorC/1 -> QuadRotor/3(motor_C)
  spdMotorA/1 -> QuadRotor/1(motor_A)
  spdMotorB/1 -> QuadRotor/2(motor_B)
  BaseTestes/1(Roll) -> Convert/1(In1)
  Convert/1(Out1) -> [OutRoll], Roll/1
  BaseTestes/2(Pitch) -> Convert1/1(In1)  "Pitch"
  BaseTestes/3(Yaw) -> Convert2/1(In1)  "Yaw"
  Convert2/1(Out1) -> [OutYaw], Yaw/1
  Convert1/1(Out1) -> [OutPitch], Pitch/1
  BaseTestes/4(Altitude) -> Convert3/1(In1)
  Convert3/1(Out1) -> [OutAlt], Altitude/1
  BaseTestes/5(X) -> [OutX], X/1
  BaseTestes/6(Y) -> [OutY], Y/1
  connections:
  BaseTestes/LConn1 -- QuadRotor/LConn1

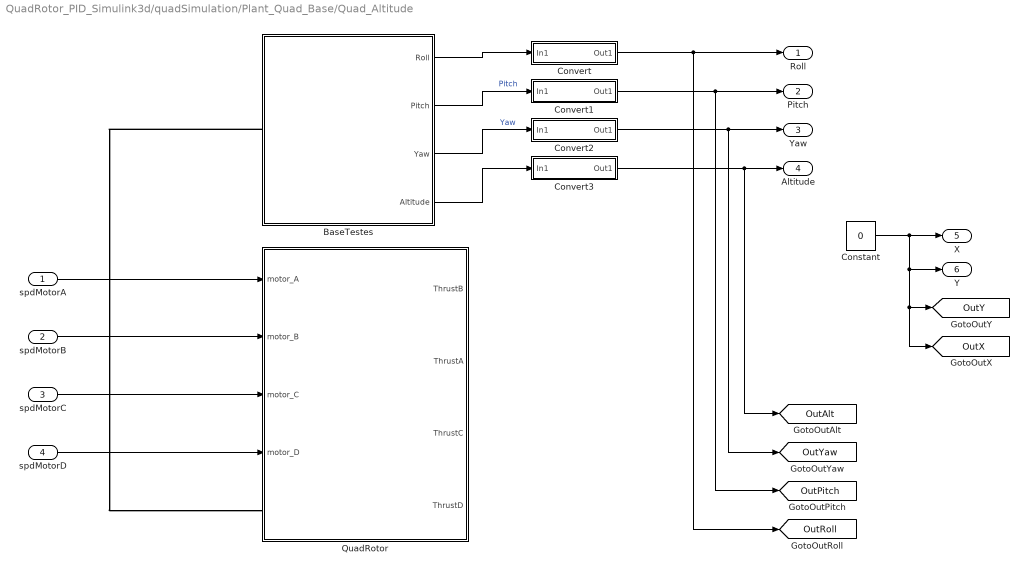
== system QuadRotor_PID_Simulink3d/quadSimulation/Plant_Quad_Base/Quad_Altitude ==
  spdMotorA : Inport
  spdMotorB : Inport  Port=2
  spdMotorC : Inport  Port=3
  spdMotorD : Inport  Port=4
  BaseTestes : Subsystem
  Constant : Constant  Value=0
  Convert : Subsystem
  Convert1 : Subsystem
  Convert2 : Subsystem
  Convert3 : Subsystem
  QuadRotor : Subsystem
  Roll : Outport
  Pitch : Outport  Port=2
  Yaw : Outport  Port=3
  Altitude : Outport  Port=4
  X : Outport  Port=5
  Y : Outport  Port=6
  tag scope: OutAlt=global, OutPitch=global, OutRoll=global, OutX=global, OutY=global, OutYaw=global
  wires:
  spdMotorD/1 -> QuadRotor/4(motor_D)
  spdMotorC/1 -> QuadRotor/3(motor_C)
  spdMotorA/1 -> QuadRotor/1(motor_A)
  spdMotorB/1 -> QuadRotor/2(motor_B)
  BaseTestes/1(Roll) -> Convert/1(In1)
  BaseTestes/2(Pitch) -> Convert1/1(In1)  "Pitch"
  BaseTestes/3(Yaw) -> Convert2/1(In1)  "Yaw"
  BaseTestes/4(Altitude) -> Convert3/1(In1)
  Convert/1(Out1) -> [OutRoll], Roll/1
  Convert2/1(Out1) -> [OutYaw], Yaw/1
  Convert1/1(Out1) -> [OutPitch], Pitch/1
  Convert3/1(Out1) -> [OutAlt], Altitude/1
  Constant/1 -> X/1, Y/1, [OutX], [OutY]
  connections:
  BaseTestes/LConn1 -- QuadRotor/LConn1

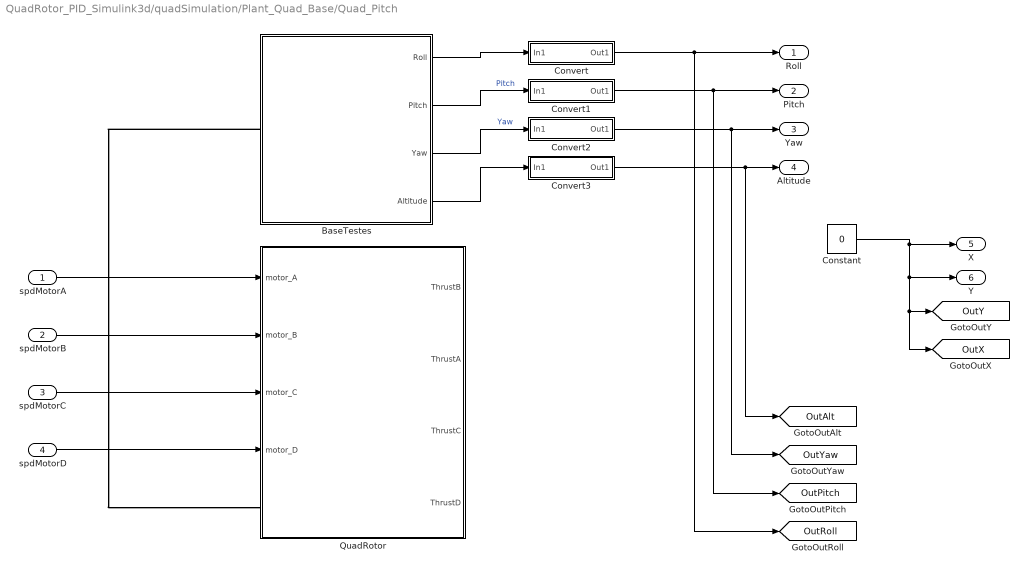
== system QuadRotor_PID_Simulink3d/quadSimulation/Plant_Quad_Base/Quad_Pitch ==
  spdMotorA : Inport
  spdMotorB : Inport  Port=2
  spdMotorC : Inport  Port=3
  spdMotorD : Inport  Port=4
  BaseTestes : Subsystem
  Constant : Constant  Value=0
  Convert : Subsystem
  Convert1 : Subsystem
  Convert2 : Subsystem
  Convert3 : Subsystem
  QuadRotor : Subsystem
  Roll : Outport
  Pitch : Outport  Port=2
  Yaw : Outport  Port=3
  Altitude : Outport  Port=4
  X : Outport  Port=5
  Y : Outport  Port=6
  tag scope: OutAlt=global, OutPitch=global, OutRoll=global, OutX=global, OutY=global, OutYaw=global
  wires:
  spdMotorD/1 -> QuadRotor/4(motor_D)
  spdMotorC/1 -> QuadRotor/3(motor_C)
  spdMotorA/1 -> QuadRotor/1(motor_A)
  spdMotorB/1 -> QuadRotor/2(motor_B)
  BaseTestes/1(Roll) -> Convert/1(In1)
  BaseTestes/2(Pitch) -> Convert1/1(In1)  "Pitch"
  BaseTestes/3(Yaw) -> Convert2/1(In1)  "Yaw"
  BaseTestes/4(Altitude) -> Convert3/1(In1)
  Convert/1(Out1) -> [OutRoll], Roll/1
  Convert2/1(Out1) -> [OutYaw], Yaw/1
  Convert1/1(Out1) -> [OutPitch], Pitch/1
  Convert3/1(Out1) -> [OutAlt], Altitude/1
  Constant/1 -> X/1, Y/1, [OutX], [OutY]
  connections:
  BaseTestes/LConn1 -- QuadRotor/LConn1

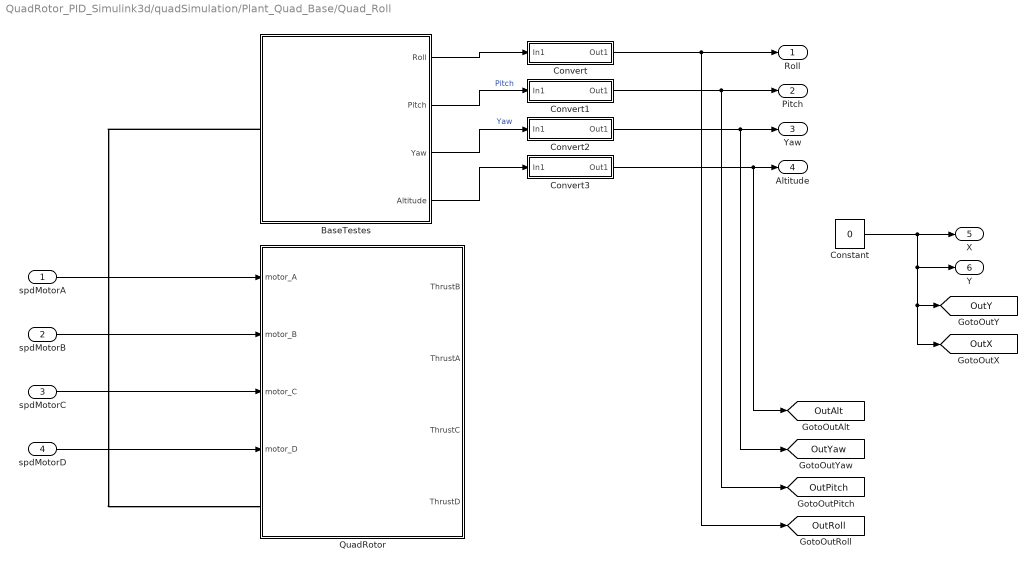
== system QuadRotor_PID_Simulink3d/quadSimulation/Plant_Quad_Base/Quad_Roll ==
  spdMotorA : Inport
  spdMotorB : Inport  Port=2
  spdMotorC : Inport  Port=3
  spdMotorD : Inport  Port=4
  BaseTestes : Subsystem
  Constant : Constant  Value=0
  Convert : Subsystem
  Convert1 : Subsystem
  Convert2 : Subsystem
  Convert3 : Subsystem
  QuadRotor : Subsystem
  Roll : Outport
  Pitch : Outport  Port=2
  Yaw : Outport  Port=3
  Altitude : Outport  Port=4
  X : Outport  Port=5
  Y : Outport  Port=6
  tag scope: OutAlt=global, OutPitch=global, OutRoll=global, OutX=global, OutY=global, OutYaw=global
  wires:
  spdMotorD/1 -> QuadRotor/4(motor_D)
  spdMotorC/1 -> QuadRotor/3(motor_C)
  spdMotorA/1 -> QuadRotor/1(motor_A)
  spdMotorB/1 -> QuadRotor/2(motor_B)
  BaseTestes/1(Roll) -> Convert/1(In1)
  BaseTestes/2(Pitch) -> Convert1/1(In1)  "Pitch"
  BaseTestes/3(Yaw) -> Convert2/1(In1)  "Yaw"
  BaseTestes/4(Altitude) -> Convert3/1(In1)
  Convert/1(Out1) -> [OutRoll], Roll/1
  Convert2/1(Out1) -> [OutYaw], Yaw/1
  Convert1/1(Out1) -> [OutPitch], Pitch/1
  Convert3/1(Out1) -> [OutAlt], Altitude/1
  Constant/1 -> X/1, Y/1, [OutX], [OutY]
  connections:
  BaseTestes/LConn1 -- QuadRotor/LConn1

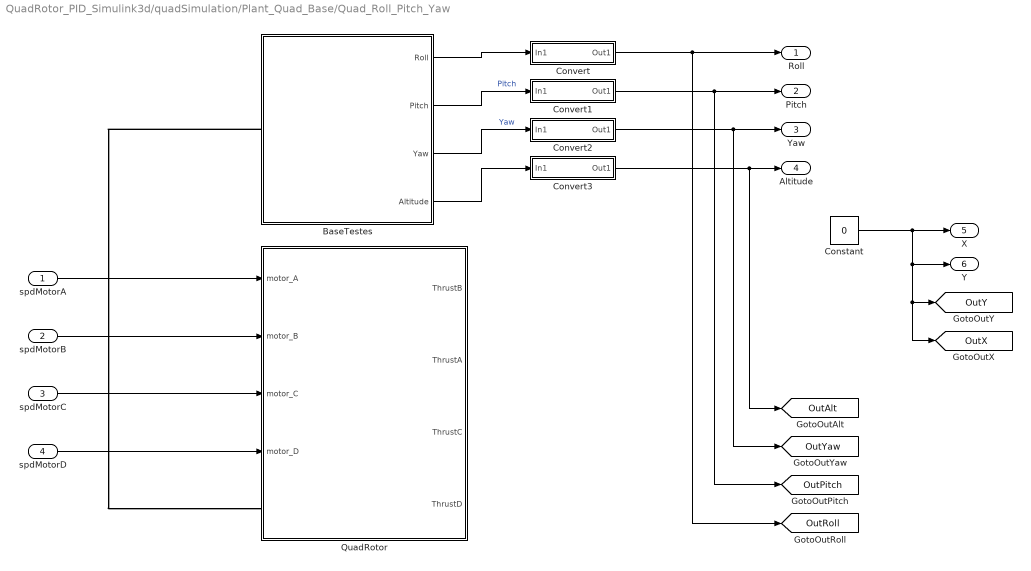
== system QuadRotor_PID_Simulink3d/quadSimulation/Plant_Quad_Base/Quad_Roll_Pitch_Yaw ==
  spdMotorA : Inport
  spdMotorB : Inport  Port=2
  spdMotorC : Inport  Port=3
  spdMotorD : Inport  Port=4
  BaseTestes : Subsystem
  Constant : Constant  Value=0
  Convert : Subsystem
  Convert1 : Subsystem
  Convert2 : Subsystem
  Convert3 : Subsystem
  QuadRotor : Subsystem
  Roll : Outport
  Pitch : Outport  Port=2
  Yaw : Outport  Port=3
  Altitude : Outport  Port=4
  X : Outport  Port=5
  Y : Outport  Port=6
  tag scope: OutAlt=global, OutPitch=global, OutRoll=global, OutX=global, OutY=global, OutYaw=global
  wires:
  spdMotorD/1 -> QuadRotor/4(motor_D)
  spdMotorC/1 -> QuadRotor/3(motor_C)
  spdMotorA/1 -> QuadRotor/1(motor_A)
  spdMotorB/1 -> QuadRotor/2(motor_B)
  BaseTestes/1(Roll) -> Convert/1(In1)
  BaseTestes/2(Pitch) -> Convert1/1(In1)  "Pitch"
  BaseTestes/3(Yaw) -> Convert2/1(In1)  "Yaw"
  BaseTestes/4(Altitude) -> Convert3/1(In1)
  Convert/1(Out1) -> [OutRoll], Roll/1
  Convert2/1(Out1) -> [OutYaw], Yaw/1
  Convert1/1(Out1) -> [OutPitch], Pitch/1
  Convert3/1(Out1) -> [OutAlt], Altitude/1
  Constant/1 -> X/1, Y/1, [OutX], [OutY]
  connections:
  BaseTestes/LConn1 -- QuadRotor/LConn1

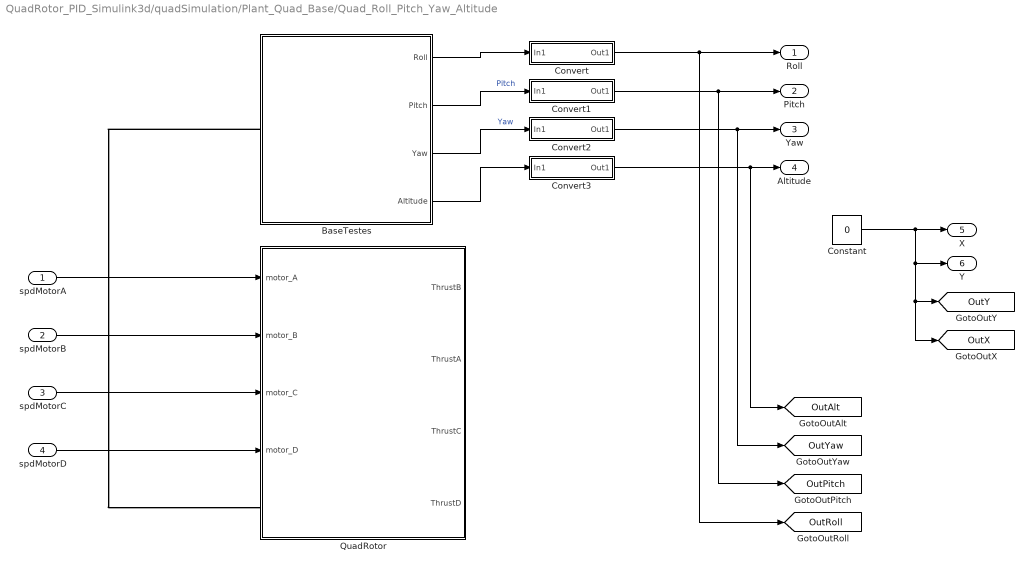
== system QuadRotor_PID_Simulink3d/quadSimulation/Plant_Quad_Base/Quad_Roll_Pitch_Yaw_Altitude ==
  spdMotorA : Inport
  spdMotorB : Inport  Port=2
  spdMotorC : Inport  Port=3
  spdMotorD : Inport  Port=4
  BaseTestes : Subsystem
  Constant : Constant  Value=0
  Convert : Subsystem
  Convert1 : Subsystem
  Convert2 : Subsystem
  Convert3 : Subsystem
  QuadRotor : Subsystem
  Roll : Outport
  Pitch : Outport  Port=2
  Yaw : Outport  Port=3
  Altitude : Outport  Port=4
  X : Outport  Port=5
  Y : Outport  Port=6
  tag scope: OutAlt=global, OutPitch=global, OutRoll=global, OutX=global, OutY=global, OutYaw=global
  wires:
  spdMotorD/1 -> QuadRotor/4(motor_D)
  spdMotorC/1 -> QuadRotor/3(motor_C)
  spdMotorA/1 -> QuadRotor/1(motor_A)
  spdMotorB/1 -> QuadRotor/2(motor_B)
  BaseTestes/1(Roll) -> Convert/1(In1)
  Convert/1(Out1) -> [OutRoll], Roll/1
  BaseTestes/2(Pitch) -> Convert1/1(In1)  "Pitch"
  BaseTestes/3(Yaw) -> Convert2/1(In1)  "Yaw"
  Convert2/1(Out1) -> [OutYaw], Yaw/1
  Convert1/1(Out1) -> [OutPitch], Pitch/1
  BaseTestes/4(Altitude) -> Convert3/1(In1)
  Convert3/1(Out1) -> [OutAlt], Altitude/1
  Constant/1 -> [OutX], [OutY], Y/1, X/1
  connections:
  BaseTestes/LConn1 -- QuadRotor/LConn1

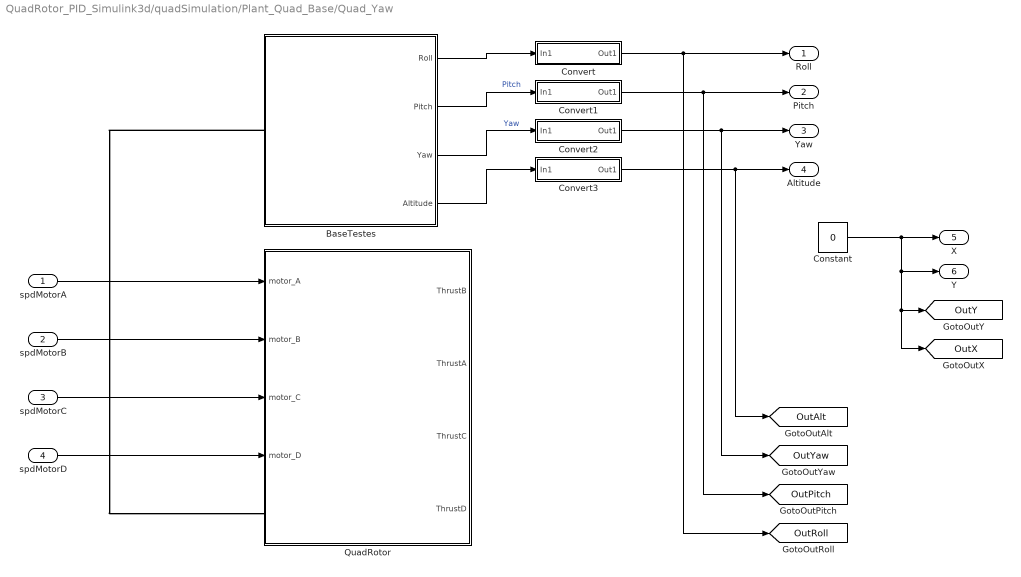
== system QuadRotor_PID_Simulink3d/quadSimulation/Plant_Quad_Base/Quad_Yaw ==
  spdMotorA : Inport
  spdMotorB : Inport  Port=2
  spdMotorC : Inport  Port=3
  spdMotorD : Inport  Port=4
  BaseTestes : Subsystem
  Constant : Constant  Value=0
  Convert : Subsystem
  Convert1 : Subsystem
  Convert2 : Subsystem
  Convert3 : Subsystem
  QuadRotor : Subsystem
  Roll : Outport
  Pitch : Outport  Port=2
  Yaw : Outport  Port=3
  Altitude : Outport  Port=4
  X : Outport  Port=5
  Y : Outport  Port=6
  tag scope: OutAlt=global, OutPitch=global, OutRoll=global, OutX=global, OutY=global, OutYaw=global
  wires:
  spdMotorD/1 -> QuadRotor/4(motor_D)
  spdMotorC/1 -> QuadRotor/3(motor_C)
  spdMotorA/1 -> QuadRotor/1(motor_A)
  spdMotorB/1 -> QuadRotor/2(motor_B)
  BaseTestes/1(Roll) -> Convert/1(In1)
  BaseTestes/2(Pitch) -> Convert1/1(In1)  "Pitch"
  BaseTestes/3(Yaw) -> Convert2/1(In1)  "Yaw"
  BaseTestes/4(Altitude) -> Convert3/1(In1)
  Convert/1(Out1) -> [OutRoll], Roll/1
  Convert2/1(Out1) -> [OutYaw], Yaw/1
  Convert1/1(Out1) -> [OutPitch], Pitch/1
  Convert3/1(Out1) -> [OutAlt], Altitude/1
  Constant/1 -> X/1, Y/1, [OutX], [OutY]
  connections:
  BaseTestes/LConn1 -- QuadRotor/LConn1

== system QuadRotor_PID_Simulink3d/quadSimulation/Plant_Quad_Base/Quad_Yaw_Altitude ==
  spdMotorA : Inport
  spdMotorB : Inport  Port=2
  spdMotorC : Inport  Port=3
  spdMotorD : Inport  Port=4
  BaseTestes : Subsystem
  Constant : Constant  Value=0
  Convert : Subsystem
  Convert1 : Subsystem
  Convert2 : Subsystem
  Convert3 : Subsystem
  QuadRotor : Subsystem
  Roll : Outport
  Pitch : Outport  Port=2
  Yaw : Outport  Port=3
  Altitude : Outport  Port=4
  X : Outport  Port=5
  Y : Outport  Port=6
  tag scope: OutAlt=global, OutPitch=global, OutRoll=global, OutX=global, OutY=global, OutYaw=global
  wires:
  spdMotorD/1 -> QuadRotor/4(motor_D)
  spdMotorC/1 -> QuadRotor/3(motor_C)
  spdMotorA/1 -> QuadRotor/1(motor_A)
  spdMotorB/1 -> QuadRotor/2(motor_B)
  BaseTestes/1(Roll) -> Convert/1(In1)
  BaseTestes/2(Pitch) -> Convert1/1(In1)  "Pitch"
  BaseTestes/3(Yaw) -> Convert2/1(In1)  "Yaw"
  BaseTestes/4(Altitude) -> Convert3/1(In1)
  Convert/1(Out1) -> [OutRoll], Roll/1
  Convert2/1(Out1) -> [OutYaw], Yaw/1
  Convert1/1(Out1) -> [OutPitch], Pitch/1
  Convert3/1(Out1) -> [OutAlt], Altitude/1
  Constant/1 -> X/1, Y/1, [OutX], [OutY]
  connections:
  BaseTestes/LConn1 -- QuadRotor/LConn1

== system QuadRotor_PID_Simulink3d/quadSimulation/Plant_Quad_Base/Quad_6Dof/BaseTestes ==
  BaseTestes : Subsystem
  ConnQuad : PMIOPort  Port=1  Side=Left
  Roll : Outport
  Pitch : Outport  Port=2
  Yaw : Outport  Port=3
  Altitude : Outport  Port=4
  X : Outport  Port=5
  Y : Outport  Port=6
  wires:
  BaseTestes/1(Roll) -> Roll/1
  BaseTestes/2(Pitch) -> Pitch/1
  BaseTestes/3(Yaw) -> Yaw/1
  BaseTestes/4(Altitude) -> Altitude/1
  BaseTestes/5(X) -> X/1
  BaseTestes/6(Y) -> Y/1
  connections:
  ConnQuad/RConn1 -- BaseTestes/LConn1

== system QuadRotor_PID_Simulink3d/quadSimulation/Plant_Quad_Base/Quad_6Dof/Convert ==
  In1 : Inport
  Add : Sum
  Constant : Constant  Value=pi/2
  ConvertAngle : MATLAB Function  TreatAsAtomicUnit=on
  Out1 : Outport
  wires:
  Constant/1 -> Add/2
  Add/1 -> ConvertAngle/1(radAngle)
  In1/1 -> Add/1
  ConvertAngle/1(AngleDeg) -> Out1/1

== system QuadRotor_PID_Simulink3d/quadSimulation/Plant_Quad_Base/Quad_6Dof/Convert1 ==
  In1 : Inport
  Add : Sum  Inputs=+-
  Constant : Constant  Value=pi/2
  ConvertAngle : MATLAB Function  TreatAsAtomicUnit=on
  Out1 : Outport
  wires:
  Constant/1 -> Add/2
  Add/1 -> ConvertAngle/1(radAngle)
  In1/1 -> Add/1
  ConvertAngle/1(AngleDeg) -> Out1/1

== system QuadRotor_PID_Simulink3d/quadSimulation/Plant_Quad_Base/Quad_6Dof/Convert2 ==
  In1 : Inport
  ConvertAngle : MATLAB Function  TreatAsAtomicUnit=on
  Out1 : Outport
  wires:
  In1/1 -> ConvertAngle/1(radAngle)
  ConvertAngle/1(AngleDeg) -> Out1/1

== system QuadRotor_PID_Simulink3d/quadSimulation/Plant_Quad_Base/Quad_6Dof/Convert3 ==
  In1 : Inport
  Gain : Gain  Gain=-1
  Out1 : Outport
  wires:
  In1/1 -> Gain/1
  Gain/1 -> Out1/1

== system QuadRotor_PID_Simulink3d/quadSimulation/Plant_Quad_Base/Quad_6Dof/QuadRotor ==
  motor_A : Inport
  motor_B : Inport  Port=2
  motor_C : Inport  Port=3
  motor_D : Inport  Port=4
  MontagemRingSuperior_1_RIGID : Subsystem
  P1 : Subsystem
  P2 : Subsystem
  P3 : Subsystem
  P4 : Subsystem
  ReferenceFrame : sm_lib/Frames and Transforms/Reference Frame  BlockFunction=simmechanics.library.frames_transforms.reference_frame
  RingInferior_1_RIGID : Subsystem
  Transform : sm_lib/Frames and Transforms/Rigid Transform  TranslationMethod=Cartesian  TranslationLengthUnit=mm  TranslationStandardAxis=+Z  TranslationStandardOffset=0  TranslationCartesianOffset=[-2.914334999999997e-16 -0.75 -2.4715275000000003e-16]  TranslationROffset=0  TranslationROffsetUnits=m  TranslationZOffset=0  TranslationZOffsetUnits=m  TranslationThetaOffset=0  TranslationThetaOffsetUnits=deg  RotationMethod=ArbitraryAxis  RotationAngleUnits=rad  RotationStandardAxis=+Z  RotationAngle=1.5707963267948963  RotationArbitraryAxis=[-1 -2.7673873760513264e-16 -7.0654160640769886e-16]  FollAlignAxisA=+X  BaseAlignAxisA=+Y  FollAlignAxisB=+Y  BaseAlignAxisB=+Z  BlockFunction=simmechanics.library.frames_transforms.rigid_transform
  Transform1 : sm_lib/Frames and Transforms/Rigid Transform  TranslationMethod=None  TranslationLengthUnit=m  TranslationStandardAxis=+Z  TranslationStandardOffset=0  TranslationCartesianOffset=[0 0 0]  TranslationROffset=0  TranslationROffsetUnits=m  TranslationZOffset=0  TranslationZOffsetUnits=m  TranslationThetaOffset=0  TranslationThetaOffsetUnits=deg  RotationMethod=None  RotationAngleUnits=deg  RotationStandardAxis=+Z  RotationAngle=0  RotationArbitraryAxis=[0 0 1]  FollAlignAxisA=+X  BaseAlignAxisA=+Y  FollAlignAxisB=+Y  BaseAlignAxisB=+Z  BlockFunction=simmechanics.library.frames_transforms.rigid_transform
  F : PMIOPort  Port=1  Side=Left
  ThrustB : Outport
  ThrustA : Outport  Port=2
  ThrustC : Outport  Port=3
  ThrustD : Outport  Port=4
  wires:
  motor_B/1 -> P1/1(SpdMotorB)
  motor_A/1 -> P2/1(SpdMotorA)
  motor_C/1 -> P3/1(SpdMotorC)
  motor_D/1 -> P4/1(SpdMotorD)
  P1/1(ThrustB) -> ThrustB/1
  P2/1(ThrustA) -> ThrustA/1
  P3/1(ThrustC) -> ThrustC/1
  P4/1(ThrustD) -> ThrustD/1
  connections:
  P2/RConn1 -- ReferenceFrame/RConn1 -- MontagemRingSuperior_1_RIGID/RConn1 -- P4/RConn1 -- P3/RConn1 -- P1/RConn1 -- Transform/LConn1 -- Transform1/LConn1
  Transform/RConn1 -- F/RConn1
  RingInferior_1_RIGID/LConn1 -- Transform1/RConn1

== system QuadRotor_PID_Simulink3d/quadSimulation/Plant_Quad_Base/Quad_Altitude/BaseTestes ==
  BaseTestes : Subsystem
  ConnQuad : PMIOPort  Port=1  Side=Left
  Roll : Outport
  Pitch : Outport  Port=2
  Yaw : Outport  Port=3
  Altitude : Outport  Port=4
  wires:
  BaseTestes/1(Roll) -> Roll/1
  BaseTestes/2(Pitch) -> Pitch/1
  BaseTestes/3(Yaw) -> Yaw/1
  BaseTestes/4(Altitude) -> Altitude/1
  connections:
  ConnQuad/RConn1 -- BaseTestes/LConn1

== system QuadRotor_PID_Simulink3d/quadSimulation/Plant_Quad_Base/Quad_Altitude/Convert ==
  In1 : Inport
  Add : Sum
  Constant : Constant  Value=0
  ConvertAngle : MATLAB Function  TreatAsAtomicUnit=on
  Out1 : Outport
  wires:
  Constant/1 -> Add/2
  Add/1 -> ConvertAngle/1(radAngle)
  In1/1 -> Add/1
  ConvertAngle/1(AngleDeg) -> Out1/1

== system QuadRotor_PID_Simulink3d/quadSimulation/Plant_Quad_Base/Quad_Altitude/Convert1 ==
  In1 : Inport
  Add : Sum  Inputs=+-
  Constant : Constant  Value=0
  ConvertAngle : MATLAB Function  TreatAsAtomicUnit=on
  Out1 : Outport
  wires:
  Constant/1 -> Add/2
  Add/1 -> ConvertAngle/1(radAngle)
  In1/1 -> Add/1
  ConvertAngle/1(AngleDeg) -> Out1/1

== system QuadRotor_PID_Simulink3d/quadSimulation/Plant_Quad_Base/Quad_Altitude/Convert2 ==
  In1 : Inport
  ConvertAngle : MATLAB Function  TreatAsAtomicUnit=on
  Out1 : Outport
  wires:
  In1/1 -> ConvertAngle/1(radAngle)
  ConvertAngle/1(AngleDeg) -> Out1/1

== system QuadRotor_PID_Simulink3d/quadSimulation/Plant_Quad_Base/Quad_Altitude/Convert3 ==
  In1 : Inport
  Gain : Gain  Gain=-1
  Out1 : Outport
  wires:
  In1/1 -> Gain/1
  Gain/1 -> Out1/1

== system QuadRotor_PID_Simulink3d/quadSimulation/Plant_Quad_Base/Quad_Altitude/QuadRotor ==
  motor_A : Inport
  motor_B : Inport  Port=2
  motor_C : Inport  Port=3
  motor_D : Inport  Port=4
  MontagemRingSuperior_1_RIGID : Subsystem
  P1 : Subsystem
  P2 : Subsystem
  P3 : Subsystem
  P4 : Subsystem
  ReferenceFrame : sm_lib/Frames and Transforms/Reference Frame  BlockFunction=simmechanics.library.frames_transforms.reference_frame
  RingInferior_1_RIGID : Subsystem
  Transform : sm_lib/Frames and Transforms/Rigid Transform  TranslationMethod=Cartesian  TranslationLengthUnit=mm  TranslationStandardAxis=+Z  TranslationStandardOffset=0  TranslationCartesianOffset=[-2.914334999999997e-16 -0.75 -2.4715275000000003e-16]  TranslationROffset=0  TranslationROffsetUnits=m  TranslationZOffset=0  TranslationZOffsetUnits=m  TranslationThetaOffset=0  TranslationThetaOffsetUnits=deg  RotationMethod=ArbitraryAxis  RotationAngleUnits=rad  RotationStandardAxis=+Z  RotationAngle=1.5707963267948963  RotationArbitraryAxis=[-1 -2.7673873760513264e-16 -7.0654160640769886e-16]  FollAlignAxisA=+X  BaseAlignAxisA=+Y  FollAlignAxisB=+Y  BaseAlignAxisB=+Z  BlockFunction=simmechanics.library.frames_transforms.rigid_transform
  Transform1 : sm_lib/Frames and Transforms/Rigid Transform  TranslationMethod=None  TranslationLengthUnit=m  TranslationStandardAxis=+Z  TranslationStandardOffset=0  TranslationCartesianOffset=[0 0 0]  TranslationROffset=0  TranslationROffsetUnits=m  TranslationZOffset=0  TranslationZOffsetUnits=m  TranslationThetaOffset=0  TranslationThetaOffsetUnits=deg  RotationMethod=None  RotationAngleUnits=deg  RotationStandardAxis=+Z  RotationAngle=0  RotationArbitraryAxis=[0 0 1]  FollAlignAxisA=+X  BaseAlignAxisA=+Y  FollAlignAxisB=+Y  BaseAlignAxisB=+Z  BlockFunction=simmechanics.library.frames_transforms.rigid_transform
  F : PMIOPort  Port=1  Side=Left
  ThrustB : Outport
  ThrustA : Outport  Port=2
  ThrustC : Outport  Port=3
  ThrustD : Outport  Port=4
  wires:
  motor_B/1 -> P1/1(SpdMotorB)
  motor_A/1 -> P2/1(SpdMotorA)
  motor_C/1 -> P3/1(SpdMotorC)
  motor_D/1 -> P4/1(SpdMotorD)
  P1/1(ThrustB) -> ThrustB/1
  P2/1(ThrustA) -> ThrustA/1
  P3/1(ThrustC) -> ThrustC/1
  P4/1(ThrustD) -> ThrustD/1
  connections:
  P2/RConn1 -- ReferenceFrame/RConn1 -- MontagemRingSuperior_1_RIGID/RConn1 -- P4/RConn1 -- P3/RConn1 -- P1/RConn1 -- Transform/LConn1 -- Transform1/LConn1
  Transform/RConn1 -- F/RConn1
  RingInferior_1_RIGID/LConn1 -- Transform1/RConn1

== system QuadRotor_PID_Simulink3d/quadSimulation/Plant_Quad_Base/Quad_Pitch/BaseTestes ==
  BaseTestes : Subsystem
  ConnQuad : PMIOPort  Port=1  Side=Left
  Roll : Outport
  Pitch : Outport  Port=2
  Yaw : Outport  Port=3
  Altitude : Outport  Port=4
  wires:
  BaseTestes/1(Roll) -> Roll/1
  BaseTestes/2(Pitch) -> Pitch/1
  BaseTestes/3(Yaw) -> Yaw/1
  BaseTestes/4(Altitude) -> Altitude/1
  connections:
  ConnQuad/RConn1 -- BaseTestes/LConn1

== system QuadRotor_PID_Simulink3d/quadSimulation/Plant_Quad_Base/Quad_Pitch/Convert ==
  In1 : Inport
  Add : Sum
  Constant : Constant  Value=pi/2
  ConvertAngle : MATLAB Function  TreatAsAtomicUnit=on
  Out1 : Outport
  wires:
  Constant/1 -> Add/2
  Add/1 -> ConvertAngle/1(radAngle)
  In1/1 -> Add/1
  ConvertAngle/1(AngleDeg) -> Out1/1

== system QuadRotor_PID_Simulink3d/quadSimulation/Plant_Quad_Base/Quad_Pitch/Convert1 ==
  In1 : Inport
  Add : Sum  Inputs=+-
  Constant : Constant  Value=pi/2
  ConvertAngle : MATLAB Function  TreatAsAtomicUnit=on
  Out1 : Outport
  wires:
  Constant/1 -> Add/2
  Add/1 -> ConvertAngle/1(radAngle)
  In1/1 -> Add/1
  ConvertAngle/1(AngleDeg) -> Out1/1

== system QuadRotor_PID_Simulink3d/quadSimulation/Plant_Quad_Base/Quad_Pitch/Convert2 ==
  In1 : Inport
  ConvertAngle : MATLAB Function  TreatAsAtomicUnit=on
  Out1 : Outport
  wires:
  In1/1 -> ConvertAngle/1(radAngle)
  ConvertAngle/1(AngleDeg) -> Out1/1

== system QuadRotor_PID_Simulink3d/quadSimulation/Plant_Quad_Base/Quad_Pitch/Convert3 ==
  In1 : Inport
  Gain : Gain  Gain=-1
  Out1 : Outport
  wires:
  In1/1 -> Gain/1
  Gain/1 -> Out1/1

== system QuadRotor_PID_Simulink3d/quadSimulation/Plant_Quad_Base/Quad_Pitch/QuadRotor ==
  motor_A : Inport
  motor_B : Inport  Port=2
  motor_C : Inport  Port=3
  motor_D : Inport  Port=4
  MontagemRingSuperior_1_RIGID : Subsystem
  P1 : Subsystem
  P2 : Subsystem
  P3 : Subsystem
  P4 : Subsystem
  ReferenceFrame : sm_lib/Frames and Transforms/Reference Frame  BlockFunction=simmechanics.library.frames_transforms.reference_frame
  RingInferior_1_RIGID : Subsystem
  Transform : sm_lib/Frames and Transforms/Rigid Transform  TranslationMethod=Cartesian  TranslationLengthUnit=mm  TranslationStandardAxis=+Z  TranslationStandardOffset=0  TranslationCartesianOffset=[-2.914334999999997e-16 -0.75 -2.4715275000000003e-16]  TranslationROffset=0  TranslationROffsetUnits=m  TranslationZOffset=0  TranslationZOffsetUnits=m  TranslationThetaOffset=0  TranslationThetaOffsetUnits=deg  RotationMethod=ArbitraryAxis  RotationAngleUnits=rad  RotationStandardAxis=+Z  RotationAngle=1.5707963267948963  RotationArbitraryAxis=[-1 -2.7673873760513264e-16 -7.0654160640769886e-16]  FollAlignAxisA=+X  BaseAlignAxisA=+Y  FollAlignAxisB=+Y  BaseAlignAxisB=+Z  BlockFunction=simmechanics.library.frames_transforms.rigid_transform
  Transform1 : sm_lib/Frames and Transforms/Rigid Transform  TranslationMethod=None  TranslationLengthUnit=m  TranslationStandardAxis=+Z  TranslationStandardOffset=0  TranslationCartesianOffset=[0 0 0]  TranslationROffset=0  TranslationROffsetUnits=m  TranslationZOffset=0  TranslationZOffsetUnits=m  TranslationThetaOffset=0  TranslationThetaOffsetUnits=deg  RotationMethod=None  RotationAngleUnits=deg  RotationStandardAxis=+Z  RotationAngle=0  RotationArbitraryAxis=[0 0 1]  FollAlignAxisA=+X  BaseAlignAxisA=+Y  FollAlignAxisB=+Y  BaseAlignAxisB=+Z  BlockFunction=simmechanics.library.frames_transforms.rigid_transform
  F : PMIOPort  Port=1  Side=Left
  ThrustB : Outport
  ThrustA : Outport  Port=2
  ThrustC : Outport  Port=3
  ThrustD : Outport  Port=4
  wires:
  motor_B/1 -> P1/1(SpdMotorB)
  motor_A/1 -> P2/1(SpdMotorA)
  motor_C/1 -> P3/1(SpdMotorC)
  motor_D/1 -> P4/1(SpdMotorD)
  P1/1(ThrustB) -> ThrustB/1
  P2/1(ThrustA) -> ThrustA/1
  P3/1(ThrustC) -> ThrustC/1
  P4/1(ThrustD) -> ThrustD/1
  connections:
  P2/RConn1 -- ReferenceFrame/RConn1 -- MontagemRingSuperior_1_RIGID/RConn1 -- P4/RConn1 -- P3/RConn1 -- P1/RConn1 -- Transform/LConn1 -- Transform1/LConn1
  Transform/RConn1 -- F/RConn1
  RingInferior_1_RIGID/LConn1 -- Transform1/RConn1

== system QuadRotor_PID_Simulink3d/quadSimulation/Plant_Quad_Base/Quad_Roll/BaseTestes ==
  BaseTestes : Subsystem
  ConnQuad : PMIOPort  Port=1  Side=Left
  Roll : Outport
  Pitch : Outport  Port=2
  Yaw : Outport  Port=3
  Altitude : Outport  Port=4
  wires:
  BaseTestes/1(Roll) -> Roll/1
  BaseTestes/2(Pitch) -> Pitch/1
  BaseTestes/3(Yaw) -> Yaw/1
  BaseTestes/4(Altitude) -> Altitude/1
  connections:
  ConnQuad/RConn1 -- BaseTestes/LConn1

== system QuadRotor_PID_Simulink3d/quadSimulation/Plant_Quad_Base/Quad_Roll/Convert ==
  In1 : Inport
  Add : Sum
  Constant : Constant  Value=pi/2
  ConvertAngle : MATLAB Function  TreatAsAtomicUnit=on
  Out1 : Outport
  wires:
  Constant/1 -> Add/2
  Add/1 -> ConvertAngle/1(radAngle)
  In1/1 -> Add/1
  ConvertAngle/1(AngleDeg) -> Out1/1
